simulink library "environment_lib"  (R2016b)
settings: Solver=ode45  StartTime=0.0  StopTime=10.0  RelTol=1e-3  EnableMultiTasking=on
undefined symbols (not defined in the file or in its folder): DT_aero_eci_Nm, DT_dipole_body_Am2, DT_grav_eci_Nm, DT_solar_eci_Nm, env_acc_eci_mps2, fsw_params, GPS_time, init_pos_eci_km, init_vel_eci_kmps, mag_vec_eci, sim_params, sun_vec_eci
libraries: bus_stubs_template x2, GPS_time_lib x1, disturbances_lib x1, time_coord_rotation_lib x1, tle2eci_coarse_lib x1
settings Model: Creator=bbarz_000  LastModifiedBy=Taylor
settings DataIOCC: LimitDataPoints=on
settings OptimizationCC: LifeSpan=inf
settings DebuggingCC: AllowSymbolicDim=off  SFUnexpectedBacktrackingDiag=warning  SFNoUnconditionalDefaultTransitionDiag=warning  SFExecutionAtInitializationDiag=none
settings GRTTargetCC: TargetLangStandard=C89/C90 (ANSI)  GeneratePreprocessorConditionals=Disable all
settings ConfigComp: CovMetricSettings=dw  CovHtmlReporting=on  CovSaveCumulativeToWorkspaceVar=on  CovSaveSingleToWorkspaceVar=on  CovExternalEMLEnable=off

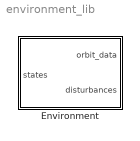
== system environment_lib ==
  Environment : Subsystem

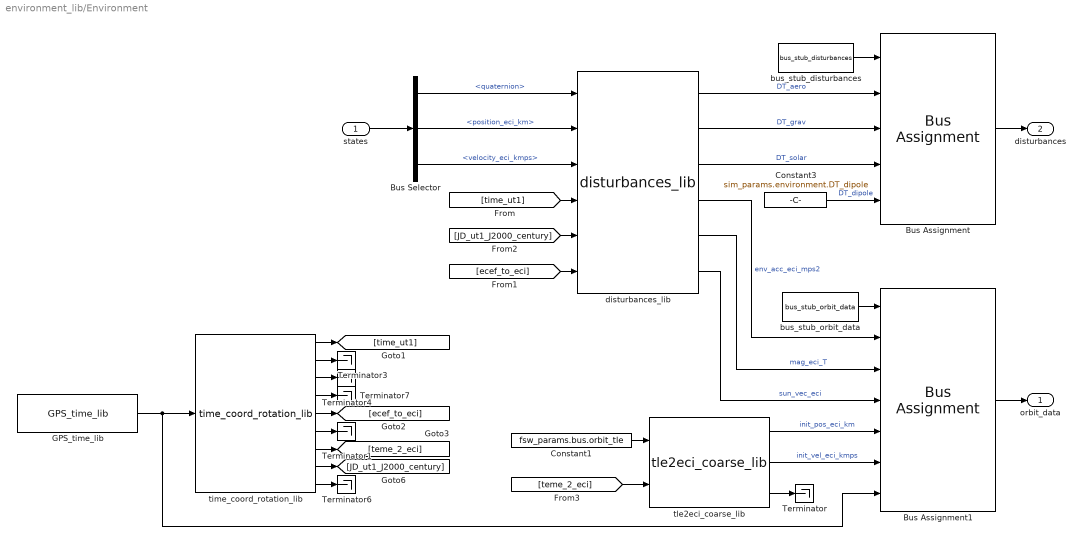
== system environment_lib/Environment ==
  states : Inport  OutDataTypeStr=Bus: states
  Bus Assignment : BusAssignment  AssignedSignals=DT_aero_eci_Nm,DT_grav_eci_Nm,DT_solar_eci_Nm,DT_dipole_body_Am2
  Bus Assignment1 : BusAssignment  AssignedSignals=env_acc_eci_mps2,mag_vec_eci,sun_vec_eci,init_pos_eci_km,init_vel_eci_kmps,GPS_time
  Bus Selector : BusSelector  OutputSignals=quaternion,position_eci_km,velocity_eci_kmps
  Constant1 : Constant  Value=fsw_params.bus.orbit_tle
  Constant3 : Constant  Value=sim_params.environment.DT_dipole
  GPS_time_lib : GPS_time_lib/GPS_time_lib
  Terminator{,1,3..4,6..7} (6 alike) : Terminator
  bus_stub_disturbances : bus_stubs_template/bus_stub_disturbances
  bus_stub_orbit_data : bus_stubs_template/bus_stub_orbit_data
  disturbances_lib : disturbances_lib/disturbances_lib
  time_coord_rotation_lib : time_coord_rotation_lib/time_coord_rotation_lib
  tle2eci_coarse_lib : tle2eci_coarse_lib/tle2eci_coarse_lib
  orbit_data : Outport
  disturbances : Outport  Port=2
  wires:
  tle2eci_coarse_lib/2 -> Bus Assignment1/6  "init_vel_eci_kmps"
  tle2eci_coarse_lib/1 -> Bus Assignment1/5  "init_pos_eci_km"
  Constant1/1 -> tle2eci_coarse_lib/1
  bus_stub_disturbances/1 -> Bus Assignment/1
  Bus Assignment/1 -> disturbances/1
  states/1 -> Bus Selector/1
  Bus Selector/1 -> disturbances_lib/1  "<quaternion>"
  Bus Selector/2 -> disturbances_lib/2  "<position_eci_km>"
  Bus Selector/3 -> disturbances_lib/3  "<velocity_eci_kmps>"
  [time_ut1] -> disturbances_lib/4
  Constant3/1 -> Bus Assignment/5  "DT_dipole"
  bus_stub_orbit_data/1 -> Bus Assignment1/1
  Bus Assignment1/1 -> orbit_data/1
  disturbances_lib/6 -> Bus Assignment1/4  "sun_vec_eci"
  [JD_ut1_J2000_century] -> disturbances_lib/5
  [ecef_to_eci] -> disturbances_lib/6
  disturbances_lib/1 -> Bus Assignment/2  "DT_aero"
  disturbances_lib/2 -> Bus Assignment/3  "DT_grav"
  disturbances_lib/3 -> Bus Assignment/4  "DT_solar"
  disturbances_lib/4 -> Bus Assignment1/2  "env_acc_eci_mps2"
  disturbances_lib/5 -> Bus Assignment1/3  "mag_eci_T"
  GPS_time_lib/1 -> Bus Assignment1/7, time_coord_rotation_lib/1
  [teme_2_eci] -> tle2eci_coarse_lib/2
  time_coord_rotation_lib/1 -> [time_ut1]
  time_coord_rotation_lib/2 -> Terminator3/1
  time_coord_rotation_lib/3 -> Terminator4/1
  time_coord_rotation_lib/4 -> Terminator7/1
  time_coord_rotation_lib/5 -> [ecef_to_eci]
  time_coord_rotation_lib/9 -> Terminator6/1
  time_coord_rotation_lib/8 -> [JD_ut1_J2000_century]
  time_coord_rotation_lib/7 -> [teme_2_eci]
  time_coord_rotation_lib/6 -> Terminator1/1
  tle2eci_coarse_lib/3 -> Terminator/1
